simulink model "lab_10_3_2018"  (R2018a)
settings: Solver=VariableStepAuto  StartTime=0.0  StopTime=10  RelTol=1e-3
undefined symbols (not defined in the file): A, C, L2, Q_2, R_2
settings Model: Creator=osini  LastModifiedBy=osini
settings DataIOCC: ReturnWorkspaceOutputs=on
settings DebuggingCC: UnconnectedInputMsg=none  UnconnectedOutputMsg=none  UnconnectedLineMsg=none  SFMachineParentedDataDiag=error
settings ModelReferenceCC: EnableRefExpFcnMdlSchedulingChecks=off
settings SFSimCC: SimUseLocalCustomCode=on
settings RTWCC: Description=Generic Real-Time Target  RTWUseLocalCustomCode=on

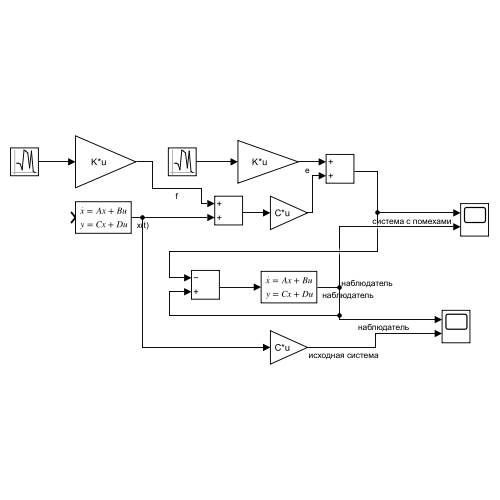
[thumbnail: Simulink's stored preview of the top-level diagram]
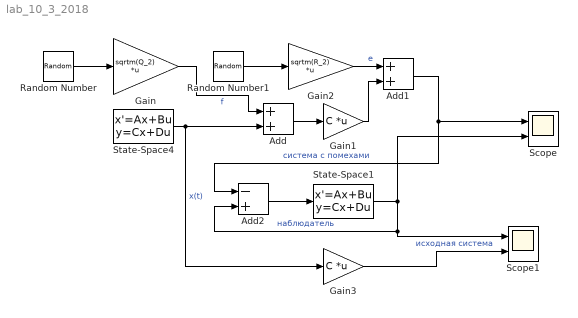
== system lab_10_3_2018 ==
  Add : Sum
  Add1 : Sum
  Add2 : Sum  Inputs=-+
  Gain : Gain  Gain=sqrtm(Q_2)  Multiplication=Matrix(K*u)
  Gain1 : Gain  Gain=C  Multiplication=Matrix(K*u)
  Gain2 : Gain  Gain=sqrtm(R_2)  Multiplication=Matrix(K*u)
  Gain3 : Gain  Gain=C  Multiplication=Matrix(K*u)
  Random Number : RandomNumber  Seed=[1;1;1;1]  SampleTime=0.001
  Random Number1 : RandomNumber  Seed=[1;1]  SampleTime=0.001
  Scope : Scope  NumInputPorts=2
  Scope1 : Scope  NumInputPorts=2
  State-Space1 : StateSpace  A=A  B=-L2  C=C  D=zeros(2,2)  InitialCondition=[2; 0; 0; 1]
  State-Space4 : StateSpace  A=A  B=zeros(4,2)  C=eye(4,4)  D=zeros(4,2)  InitialCondition=1
  wires:
  Random Number/1 -> Gain/1
  State-Space4/1 -> Gain3/1, Add/2  "x(t)"
  Gain/1 -> Add/1  "f"
  Add/1 -> Gain1/1
  Gain1/1 -> Add1/2
  Gain2/1 -> Add1/1  "e"
  Random Number1/1 -> Gain2/1
  Add1/1 -> Add2/1, Scope/1  "система с помехами"
  Add2/1 -> State-Space1/1
  State-Space1/1 -> Scope/2, Scope1/1, Add2/2  "наблюдатель"
  Gain3/1 -> Scope1/2  "исходная система"
